simulink model "PIL_NO_RPI_new"  (R2021a)
settings: Solver=FixedStepAuto  StartTime=0.0  StopTime=60  FixedStep=0.001  RelTol=1e-3  EnableMultiTasking=on
values from neighbouring files (symbols this model uses):
  den_lpf_d = den_lpf20    [Mainframe_init.m]    (also in load_autopilot.m)
  Enable_Gyros = 0    [Mainframe_init.m]
  Enable_INS = 0    [Mainframe_init.m]
  num_lpf_d = num_lpf20    [Mainframe_init.m]    (also in load_autopilot.m)
undefined symbols (not defined in the file or in its folder): act_dmp, act_omega, Actuator, Aerodynamics, aMode, Autopilot, AUX, c_b_WGS, c_be, c_flat, c_grav, c_h_geop0, c_h_geope, c_pa0, c_pe, c_r0, c_rot, c_rsma, c_Tmp0, d_siB_0, d_siB_max, d_siB_min, dd_siB_max, dd_siB_min, dev, DiscIntNeverNeededParam, e_pa, e_Tmp, fin_maxrate, flag_I_act_switch, flag_I_aero_switch, flag_I_flat, flag_I_gravity_switch, flag_I_rot, h_bkpts_m, hcr, HIL_Data, JMMM_0, JMMM_e, JSPB_e, Ki_phi_vec, Kp_p_vec, Kp_phi_vec, lat_0, lon_0, Mass_Props, mB_0, mM_0, mM_e, National_Instruments, Newton, p, pBII_0, PCIe, phi, pMPB, pNPB, propellant_kg, prp_FBPB, prp_mdot ... (+40)
libraries: simulink x32, simulink_extras x23, aerolibcommonsys x4, pil_lib x2, custom_blocks x1, px4lib x1, sldrtlib x1, aerolibnav x1
(part 2 of 16)

== system PIL_NO_RPI_new/Servos1/Emulated Servos ==
  FCC Data : Inport
  Bus Creator : BusCreator  Inputs=4
  Bus Selector : BusSelector  OutputSignals=Control Surface Cmd.Fin_1_Cmd_rad,Control Surface Cmd.Fin_2_Cmd_rad,Control Surface Cmd.Fin_3_Cmd_rad,Control Surface Cmd.Fin_4_Cmd_rad
  Transfer Fcn{1..4} (4 alike) : TransferFcn  Numerator=33770  Denominator=[1 395.7 33770]
  Fin Deflections : Outport
  wires:
  FCC Data/1 -> Bus Selector/1
  Bus Selector/1 -> Transfer Fcn1/1  "<Fin_1_Cmd_rad>"
  Bus Selector/2 -> Transfer Fcn2/1  "<Fin_2_Cmd_rad>"
  Bus Selector/3 -> Transfer Fcn3/1  "<Fin_3_Cmd_rad>"
  Bus Selector/4 -> Transfer Fcn4/1  "<Fin_4_Cmd_rad>"
  Bus Creator/1 -> Fin Deflections/1
  Transfer Fcn1/1 -> Bus Creator/1  "Fin_1"
  Transfer Fcn2/1 -> Bus Creator/2  "Fin_2"
  Transfer Fcn3/1 -> Bus Creator/3  "Fin_3"
  Transfer Fcn4/1 -> Bus Creator/4  "Fin_4"

== system PIL_NO_RPI_new/Servos1/Real Servos ==
  FCC Data : Inport
  Bus Creator : BusCreator  Inputs=4
  Demux : Demux
  Encoder Input : sldrtlib/Encoder Input  SampleTime=0.001  MaxMissedTicks=10  ShowMissedTicks=off  YieldWhenWaiting=off  DrvName=National_Instruments/PCIe-6321  DrvAddress=4294967295  DrvOptions=[0 0 0 2 2 2 2]  Channels=1:4  QuadMode=3  IndexPulse=1  InputFilter=Inf  DataType=1
      settings: AttributesFormatString=National Instruments\nPCIe-6321 [auto]
  Reset Encoders : Subsystem
  Terminator : Terminator
  Ticks to rads : Gain  Gain=2*pi/4096
  Fin Deflections : Outport
  wires:
  Encoder Input/1 -> Ticks to rads/1
  FCC Data/1 -> Terminator/1
  Bus Creator/1 -> Fin Deflections/1
  Demux/3 -> Bus Creator/3  "Fin_3"
  Demux/2 -> Bus Creator/2  "Fin_2"
  Demux/1 -> Bus Creator/1  "Fin_1"
  Demux/4 -> Bus Creator/4  "Fin_4"
  [HIL_Ready] -> Reset Encoders/1(Reset Encoders)
  Ticks to rads/1 -> Reset Encoders/2(Encoder Readings)
  Reset Encoders/1(Fin Angles) -> Demux/1

== system PIL_NO_RPI_new/Virtual IMU/Gravity Vector ==
  Phi : Inport
  Theta : Inport  Port=2
  Cos : Trigonometry
  Cos1 : Trigonometry
  Cos2 : Trigonometry  Operator=cos
  Cos3 : Trigonometry  Operator=cos
  Multiply : Gain  Gain=9.81
  Multiply1 : Gain  Gain=9.81
  Multiply2 : Gain  Gain=-9.81
  Product : Product
  Product1 : Product
  Vector Concatenate1 : Concatenate  NumInputs=3
  g : Outport
  wires:
  Vector Concatenate1/1 -> g/1
  Cos/1 -> Multiply2/1
  Product/1 -> Multiply/1
  Cos1/1 -> Product/1
  Theta/1 -> Cos/1, Cos2/1
  Multiply/1 -> Vector Concatenate1/2
  Phi/1 -> Cos3/1, Cos1/1
  Product1/1 -> Multiply1/1
  Multiply1/1 -> Vector Concatenate1/3
  Multiply2/1 -> Vector Concatenate1/1
  Cos2/1 -> Product1/1, Product/2
  Cos3/1 -> Product1/2

== system PIL_NO_RPI_new/Flight Control Computer1/Communication Delay - 7ms/Triggered Subsystem ==
  In1 : Inport
  Trigger : TriggerPort  VariantControl=Variant
  Out1 : Outport
  wires:
  In1/1 -> Out1/1

== system PIL_NO_RPI_new/Flight Control Computer1/Communication Delay - 7ms1/Triggered Subsystem ==
  In1 : Inport
  Trigger : TriggerPort  VariantControl=Variant
  Out1 : Outport
  wires:
  In1/1 -> Out1/1

== system PIL_NO_RPI_new/Flight Control Computer1/PixBlock/Emulated Pixhawk1 ==
  Serial In : Inport
  Trigger : TriggerPort  VariantControl=Variant  PortDimensions=1
  Autopilot : Subsystem
  Convert to Bus : Subsystem
  Convert to Vector : Subsystem
  Fin Allocation : Subsystem
  IMU - Merge : Subsystem
  Inertial Navigation System : Subsystem
  Real Gyro : Subsystem
  Servo Commands : Subsystem  Commented=on
  Terminator : Terminator
  Zero : Constant  Value=0  OutDataTypeStr=Inherit: Inherit via back propagation
  Serial Out : Outport
  tag scope: Heartbeat=global
  wires:
  [Real_Gyro_Data] -> Convert to Vector/4(Real Gyro Data)
  Convert to Bus/2(Ext. Commands) -> [Ext_Cmd]
  Autopilot/1(Attitude_Commands) -> Fin Allocation/1(Attitude Cmd)  "ATT_Cmd"
  Convert to Bus/3(Enable INS Flag) -> Inertial Navigation System/1(Enable INS Flag)
  Inertial Navigation System/1(INS Data) -> [INS_Data]
  Zero/1 -> Convert to Vector/5(Debug Port)
  [Ext_Cmd] -> Autopilot/1(Cmd)
  [Heartbeat] -> Convert to Vector/2(Heartbeat)
  [IMU_Data] -> Autopilot/2(IMU Data)
  [INS_Data] -> Autopilot/3(INS Data)
  Convert to Bus/6(Virtual IMU Data) -> Real Gyro/1(HIL Gyro), IMU - Merge/1(HIL IMU)
  IMU - Merge/1(IMU Data) -> [IMU_Data], Inertial Navigation System/3(IMU Data)
  Convert to Vector/1(To HIL) -> Serial Out/1
  Fin Allocation/1(Fin Cmd) -> Servo Commands/1(Fin Cmd), Convert to Vector/1(Fin Deflections)
  Serial In/1 -> Convert to Bus/1(Input)
  [INS_Data] -> Convert to Vector/3(INS Data)
  Convert to Bus/4(Missile States) -> Inertial Navigation System/2(Missile States)
  Convert to Bus/1(Heartbeat) -> [Heartbeat]
  Convert to Bus/5(Real Gyros Flag) -> Terminator/1
  Real Gyro/1(Gyro Data) -> [Real_Gyro_Data]

== system PIL_NO_RPI_new/Flight Control Computer1/PixBlock1/__InputSSForSFun__ ==
  Serial In : Inport
  __UniqueOutportName__1__ : Outport
  wires:
  Serial In/1 -> __UniqueOutportName__1__/1

== system PIL_NO_RPI_new/Flight Control Computer1/PixBlock1/__OutputSSForSFun__ ==
  __UniqueInportName__1__ : Inport
  Serial Out : Outport
  wires:
  __UniqueInportName__1__/1 -> Serial Out/1

== system PIL_NO_RPI_new/Flight Control Computer1/Send to FCC/Heartbeat Counter ==
  note: Starting the heartbeat at negative values prevents unwanted FCC behaviour on startup
  Cast To Double14 : DataTypeConversion  OutDataTypeStr=single
  Heartbeat : simulink/Sources/Counter Free-Running  NumBits=16  tsamp=-1
  Subtract : Sum  Inputs=+-
  Zero : Constant  Value=1000  OutDataTypeStr=Inherit: Inherit via back propagation
  Out1 : Outport
  wires:
  Heartbeat/1 -> Cast To Double14/1
  Zero/1 -> Subtract/2
  Cast To Double14/1 -> Subtract/1  "send"
  Subtract/1 -> Out1/1

== system PIL_NO_RPI_new/Flight Control Computer2/Communication Delay - 7ms/Triggered Subsystem ==
  In1 : Inport
  Trigger : TriggerPort  VariantControl=Variant
  Out1 : Outport
  wires:
  In1/1 -> Out1/1

== system PIL_NO_RPI_new/Flight Control Computer2/Communication Delay - 7ms1/Triggered Subsystem ==
  In1 : Inport
  Trigger : TriggerPort  VariantControl=Variant
  Out1 : Outport
  wires:
  In1/1 -> Out1/1

== system PIL_NO_RPI_new/Flight Control Computer2/Communication Delay - 7ms2/Triggered Subsystem ==
  In1 : Inport
  Trigger : TriggerPort  VariantControl=Variant
  Out1 : Outport
  wires:
  In1/1 -> Out1/1

== system PIL_NO_RPI_new/Flight Control Computer2/Pixhawk1/FCC Logic1 ==
  Ext. Commands : Inport
  FDM States : Inport  Port=2
  ALT : Inport  Port=3
  Control : Subsystem
  Fin Allocation : Subsystem
  variable switch : Subsystem
  Fin Deflections : Outport
  wires:
  Fin Allocation/1(siB_cmd) -> Fin Deflections/1
  Control/1(Attitude_Commands) -> Fin Allocation/1(Input1)  "ATT_Cmd"
  Ext. Commands/1 -> Control/1(cmd)
  variable switch/1(State Bus) -> Control/2(states)
  FDM States/1 -> variable switch/1(Simulation States)
  ALT/1 -> Control/3(ALT)

== system PIL_NO_RPI_new/Flight Control Computer2/Pixhawk1/Send to HIL ==
  Fin Deflections1 : Inport
  Heartbeat1 : Inport  Port=2
  Debug Port1 : Inport  Port=3
  Cast To Single : DataTypeConversion  OutDataTypeStr=single
  Cast To Single3 : DataTypeConversion  OutDataTypeStr=single
  Cast To Single4 : DataTypeConversion  OutDataTypeStr=single
  Demux1 : Demux
  Vector Concatenate1 : Concatenate  NumInputs=6
  control_allocation1 : Subsystem
  Data Out : Outport
  wires:
  Cast To Single/1 -> Data Out/1
  Heartbeat1/1 -> Vector Concatenate1/1
  control_allocation1/1(siB_cmd) -> Cast To Single4/1
  Fin Deflections1/1 -> Cast To Single3/1
  Cast To Single3/1 -> control_allocation1/1(fin_cmd)
  Cast To Single4/1 -> Demux1/1
  Demux1/1 -> Vector Concatenate1/2  "siB_cmd_1"
  Demux1/2 -> Vector Concatenate1/3  "siB_cmd_2"
  Demux1/3 -> Vector Concatenate1/4  "siB_cmd_3"
  Demux1/4 -> Vector Concatenate1/5  "siB_cmd_4"
  Debug Port1/1 -> Vector Concatenate1/6
  Vector Concatenate1/1 -> Cast To Single/1

== system PIL_NO_RPI_new/Flight Control Computer2/Pixhawk1/data2bus ==
  raw_data : Inport  OutDataTypeStr=single
  Bus Creator : BusCreator  Inputs=9
  Bus Creator1 : BusCreator  Inputs=1
  Demux : Demux  Outputs=13
  Ext. Commands : Outport  OutDataTypeStr=single
  FDM States : Outport  Port=2  OutDataTypeStr=single
  Heartbeat : Outport  Port=3
  FCC Enabled : Outport  Port=4
  Use Sim States : Outport  Port=5
  wires:
  Demux/10 -> Bus Creator/7  "u"
  Demux/3 -> Use Sim States/1  "Use Sim States"
  Demux/2 -> Heartbeat/1  "Hearbeat"
  Demux/8 -> Bus Creator/5  "q"
  Demux/4 -> Bus Creator/1  "phi"
  Demux/5 -> Bus Creator/2  "theta"
  Demux/7 -> Bus Creator/4  "p"
  Demux/9 -> Bus Creator/6  "r"
  Demux/6 -> Bus Creator/3  "psi"
  Demux/13 -> Bus Creator1/1  "phi_cmd"
  Demux/12 -> Bus Creator/9  "w"
  Demux/11 -> Bus Creator/8  "v"
  raw_data/1 -> Demux/1
  Bus Creator/1 -> FDM States/1
  Bus Creator1/1 -> Ext. Commands/1
  Demux/1 -> FCC Enabled/1  "EnableFCC"

== system PIL_NO_RPI_new/Flight Control Computer2/Pixhawk2/__InputSSForSFun__ ==
  Input Data : Inport
  "ALT " : Inport  Port=2
  __UniqueOutportName__1__ : Outport
  __UniqueOutportName__2__ : Outport  Port=2
  wires:
  "ALT "/1 -> __UniqueOutportName__2__/1
  Input Data/1 -> __UniqueOutportName__1__/1

== system PIL_NO_RPI_new/Flight Control Computer2/Pixhawk2/__OutputSSForSFun__ ==
  __UniqueInportName__1__ : Inport
  Output Data : Outport
  wires:
  __UniqueInportName__1__/1 -> Output Data/1

== system PIL_NO_RPI_new/Flight Control Computer2/Send to Pixhawk/HeartBeat ==
  note: Starting the heartbeat at negative values prevents unwanted FCC behaviour on startup
  Cast To Double14 : DataTypeConversion  OutDataTypeStr=single
  Heartbeat : simulink/Sources/Counter Free-Running  NumBits=16  tsamp=-1
  Subtract : Sum  Inputs=+-
  Zero : Constant  Value=1000  OutDataTypeStr=Inherit: Inherit via back propagation
  Out1 : Outport
  wires:
  Heartbeat/1 -> Cast To Double14/1
  Zero/1 -> Subtract/2
  Cast To Double14/1 -> Subtract/1  "send"
  Subtract/1 -> Out1/1

== system PIL_NO_RPI_new/Flight Control Computer2/Send to Pixhawk/State Mixer ==
  States : Inport
  Bus Selector : BusSelector  OutputSignals=Attitude_States.ATT_Euler.Phi_rad,Attitude_States.ATT_Euler.Theta_rad,Attitude_States.ATT_Euler.Psi_rad,Rotation_States.p_radDs,Rotation_States.q_radDs,Rotation_States.r_radDs,Translation_States.u_mDs,Translation_States.v_mDs,Translation_States.w_mDs
  Phi_rad : Outport
  Theta_rad : Outport  Port=2
  Psi_rad : Outport  Port=3
  p_radDs : Outport  Port=4
  q_radDs : Outport  Port=5
  r_radDs : Outport  Port=6
  u_mDs : Outport  Port=7
  v_mDs : Outport  Port=8
  w_mDs : Outport  Port=9
  wires:
  Bus Selector/3 -> Psi_rad/1  "<Psi_rad>"
  Bus Selector/9 -> w_mDs/1  "<w_mDs>"
  Bus Selector/1 -> Phi_rad/1  "<Phi_rad>"
  Bus Selector/5 -> q_radDs/1  "<q_radDs>"
  Bus Selector/7 -> u_mDs/1  "<u_mDs>"
  Bus Selector/6 -> r_radDs/1  "<r_radDs>"
  Bus Selector/2 -> Theta_rad/1  "<Theta_rad>"
  States/1 -> Bus Selector/1
  Bus Selector/8 -> v_mDs/1  "<v_mDs>"
  Bus Selector/4 -> p_radDs/1  "<p_radDs>"

== system PIL_NO_RPI_new/Flight Gear Simulator/Flight Simulator On/Flat Earth to LLA ==
  Xe : Inport  Unit=m
  ground height : Inport  Port=2  Unit=m
  Disallow CGS : UnitConfiguration  UnitSystemsStr=English,SI,SI (extended)  AllowAllUnitSystems=off
  LatLong wrap : Subsystem
      mask init:
      | aeroicon('aeroblk')
      mask Display:
      | port_label('input',1,'[\mu l]','texmode','on')
      | port_label('output',1,'[\mu l]_{wrap}','texmode','on')
  LatLong wrap1 : Subsystem
      mask init:
      | aeroicon('aeroblk')
      mask Display:
      | port_label('input',1,'[\mu l]','texmode','on')
      | port_label('output',1,'[\mu l]_{wrap}','texmode','on')
  LongLat_offset : Subsystem
  Sel1 : Selector  InputPortWidth=3  IndexOptions=Index vector (dialog)  Indices=[1,2]  OutputSizes=1
  Sel2 : Selector  InputPortWidth=3  IndexOptions=Index vector (dialog)  Indices=3  OutputSizes=1
  Sum : Sum  Inputs=|++
  Sum1 : Sum  Inputs=-+
  "Xe " : InportShadow  Unit=m
  Ze2height : UnaryMinus
  initial_latg : Selector  InputPortWidth=2  IndexOptions=Index vector (dialog)  Indices=[1]  OutputSizes=1
  initial_pos : Constant  Value=LL0
  pos_deg : Subsystem
  mu l : Outport  Unit=deg  VectorParamsAs1DForOutWhenUnconnected=off
  h : Outport  Port=2  Unit=m  VectorParamsAs1DForOutWhenUnconnected=off
  wires:
  pos_deg/1(out) -> Sum/1
  LongLat_offset/1(DeltaLL_rad) -> pos_deg/1(in)
  LatLong wrap1/1(Lat/Long wrapped) -> initial_latg/1, Sum/2
  initial_pos/1 -> LatLong wrap1/1(LatLong)
  LatLong wrap/1(Lat/Long wrapped) -> mu l/1
  initial_latg/1 -> LongLat_offset/2(mu)
  "Xe "/1 -> Sel2/1
  Sel1/1 -> LongLat_offset/1(XY)
  ground height/1 -> Sum1/1
  Sum1/1 -> h/1
  Ze2height/1 -> Sum1/2  "alt"
  Sel2/1 -> Ze2height/1
  Sum/1 -> LatLong wrap/1(LatLong)
  Xe/1 -> Sel1/1

== system PIL_NO_RPI_new/Flight Gear Simulator/Flight Simulator On/FlightGear Preconfigured 6DoF Animation ==
  In1 : Inport
  Angle Conversion : Subsystem
  Angle Conversion1 : Subsystem
  Demux : Demux  Outputs=6
  Pack net_fdm Packet for FlightGear : S-Function  FunctionName=saerofgpacknetfdm  Parameters=packetVersion, 'on','off','off','off','off','off', SampleTime  SFunctionDeploymentMode=off  EnableBusSupport=off
  PacketSize : Constant  Value=408
  Rate Transition : RateTransition  Integrity=off  Deterministic=off  OutPortSampleTime=SampleTime
  Simulation Pace : S-Function  FunctionName=saeroclockpacer  Parameters=SimulationPace,SleepMode,OutputPaceError,SampleTime  SFunctionDeploymentMode=off  EnableBusSupport=off  mask(Simulation Pace){SimulationPace=1, SleepMode=MATLAB Thread, OutputPaceError=off, SampleTime=SampleTime}
      mask prompts: SimulationPace "aeroblks:aeroblkanimutils:blockSimulationPaceParamSimulationpacesimsecperclocksec"; SleepMode "aeroblks:aeroblkanimutils:blockSimulationPaceParamSleepmode"; OutputPaceError "aeroblks:aeroblkanimutils:blockSimulationPaceParamOutputpaceerrorsec"; SampleTime "aeroblks:aeroblkanimutils:blockSimulationPaceParamSampletime1forinherited"
      mask help: aeroblks:aeroblkanimutils:blockSimulationPaceDesc
      mask init:
      | aeroicon('aeroblkpacer');
      settings: AttributesFormatString=%<SimulationPace> sec/sec
      mask Help: eval('asbhelp');
      mask TypeOptions SleepMode: aeroblks:aeroblkanimutils:blockSimulationPaceParamComboOff | aeroblks:aeroblkanimutils:blockSimulationPaceParamComboMATLABThread | aeroblks:aeroblkanimutils:blockSimulationPaceParamComboBusyWait | aeroblks:aeroblkanimutils:blockSimulationPaceParamComboAuto
      mask DialogControl SimulationPace Prompt: Simulation pace (sim sec per clock sec):
      mask DialogControl SleepMode Prompt: Sleep mode:
      mask DialogControl OutputPaceError Prompt: Output pace error (sec)
      mask DialogControl SampleTime Prompt: Sample time (-1 for inherited):
      mask Display:
      | text(0.5,0.60,'Set','horizontalAlignment','center');
      | text(0.5,0.40,'Pace','horizontalAlignment','center');
  UDP Send : S-Function  FunctionName=saerofgsend  Parameters=DestinationIpAddress,DestinationPort,-1,SampleTime,0  SFunctionDeploymentMode=off  EnableBusSupport=off
  Unit Sys : UnitConfiguration  UnitSystemsStr=SI,SI (extended)  AllowAllUnitSystems=off
  toSingle1 : DataTypeConversion  OutDataTypeStr=single
  toSingle2 : DataTypeConversion  OutDataTypeStr=single
  toSingle3 : DataTypeConversion  OutDataTypeStr=single
  wires:
  Angle Conversion1/1(out) -> Pack net_fdm Packet for FlightGear/2
  Angle Conversion/1(out) -> Pack net_fdm Packet for FlightGear/1
  Rate Transition/1 -> Demux/1
  toSingle3/1 -> Pack net_fdm Packet for FlightGear/6
  toSingle2/1 -> Pack net_fdm Packet for FlightGear/5
  toSingle1/1 -> Pack net_fdm Packet for FlightGear/4
  Pack net_fdm Packet for FlightGear/1 -> UDP Send/1
  In1/1 -> Rate Transition/1
  Demux/1 -> Angle Conversion/1(in)
  Demux/2 -> Angle Conversion1/1(in)
  Demux/3 -> Pack net_fdm Packet for FlightGear/3
  Demux/4 -> toSingle1/1
  Demux/5 -> toSingle2/1
  Demux/6 -> toSingle3/1
  PacketSize/1 -> UDP Send/2

== system PIL_NO_RPI_new/Flight Gear Simulator/Flight Simulator On/FlightGear1 ==

== system PIL_NO_RPI_new/Non-linear Flight Dynamic Model1/Environment/Enabled Subsystem1 ==
  Enable : EnablePort
  Digital Clock : DigitalClock  SampleTime=-1
  CalibrationTime : Outport  InitialOutput=0
  wires:
  Digital Clock/1 -> CalibrationTime/1

== system PIL_NO_RPI_new/Non-linear Flight Dynamic Model1/Environment/atm_dynamic ==
  Add : Sum
  Add1 : Sum
  Bus Creator : BusCreator  Inputs=1
  Constant1 : Constant  Value=0
  Vector Concatenate : Concatenate  NumInputs=3
  course_angle_uncertainty : Constant  Value=0
  course_angle_wind : Constant  Value=0
  trafo_around_z_axis : Subsystem  mask(Transformation um z-Achse){}
      mask help: Dieser Block transformiert einen Vektor vec1 durch eine Drehung des Referenzkoordinatensystems um die z-Achse und um den Winkel gamma (in rad) in den Vektor vec2
      mask Help:
      | Name:
      | 
      |    trafo_around_z_axis
      | 
      | Beschreibung:
      | 
      |    Dieser Block transformiert einen Vektor vec1 durch eine Drehung des
      |    Referenzkoordinatensystems um die z-Achse und um den Winkel gamma
      |    (in rad) in den Vektor vec2
      | 
      | Inputs   [dimension]  [data type] [unit]:
      | 
      |     vec1    [3] [double] [-]
      |     gamma   [1] [double] [rad]
      | 
      | Outputs  [dimension]  [data type] [unit]:
      | 
      |     vec2  [3] [double] [-]
  vWW : Constant  Value=0
  vWW_uncertainty : Constant  Value=0
  vWEG : Outport  VectorParamsAs1DForOutWhenUnconnected=off
  wires:
  Bus Creator/1 -> vWEG/1  "atm_dyn_bus"
  trafo_around_z_axis/1(vec2) -> Bus Creator/1  "vWEG"
  Add1/1 -> Vector Concatenate/1
  course_angle_uncertainty/1 -> Add/2
  Constant1/1 -> Vector Concatenate/2, Vector Concatenate/3
  vWW/1 -> Add1/2
  Vector Concatenate/1 -> trafo_around_z_axis/1(vec1)
  Add/1 -> trafo_around_z_axis/2(gamma)
  vWW_uncertainty/1 -> Add1/1
  course_angle_wind/1 -> Add/1

== system PIL_NO_RPI_new/Non-linear Flight Dynamic Model1/Extract States/Assemble_States_Bus1 ==
  Translation_States : Inport
  Rotation_States : Inport  Port=2
  Translation_States_Dot : Inport  Port=3
  Rotation_States_Dot : Inport  Port=4
  Attitude_States : Inport  Port=5
  POS_NED : Inport  Port=6
  POS_NED_dot : Inport  Port=7
  Bus Creator{1,4..6,8,12..13} (7 alike) : BusCreator  Inputs=3
  Bus Creator3 : BusCreator  Inputs=7
  Bus Creator7 : BusCreator  Inputs=2
  Bus Creator9 : BusCreator  Inputs=4
  Demux : Demux
  Demux{1..7} (7 alike) : Demux  Outputs=3
  Rotation Angles to Quaternions : Subsystem  mask(Ang2Quat){rotationOrder=ZYX, aMode=aMode}
      mask prompts: rotationOrder "shared_aeroblks:sharedaeroblktransform:blockAng2QuatParamRotationOrder"
      mask help: shared_aeroblks:sharedaeroblktransform:blockAng2QuatDesc
      mask init:
      | if aerosharedtest(gcb)
      |     ports=aerosharedicon('sharedang2quat');
      | else
      |     ports=sharedautoicon('sharedang2quat');
      | end
      settings: AttributesFormatString=Rotation Order: %<rotationOrder>
      mask Help: eval('if license(''test'',''Aerospace_Blockset'')aerosharedhelp(''rotation_angles_to_quaternions'');elseif license(''test'',''Powertrain_Blockset'')sharedautohelp(''rotation_angles_to_quaternions'');end')
      mask TypeOptions rotationOrder: shared_aeroblks:sharedaeroblktransform:blockParamComboZYX | shared_aeroblks:sharedaeroblktransform:blockParamComboZYZ | shared_aeroblks:sharedaeroblktransform:blockParamComboZXY | shared_aeroblks:sharedaeroblktransform:blockParamComboZXZ | shared_aeroblks:sharedaeroblktransform:blockParamComboYXZ | shared_aeroblks:sharedaeroblktransform:blockParamComboYXY | shared_aeroblks:sharedaeroblktransform:blockParamComboYZX | shared_aeroblks:sharedaeroblktransform:blockParamComboYZY | shared_aeroblks:sharedaeroblktransform:blockParamComboXYZ | shared_aeroblks:sharedaeroblktransform:blockParamComboXYX | shared_aeroblks:sharedaeroblktransform:blockParamComboXZY | shared_aeroblks:sharedaeroblktransform:blockParamComboXZX
      mask DialogControl rotationOrder Prompt: Rotation order:
      mask Display:
      | port_label('input',1,'[R_1,R_2,R_3]','texmode','on')
      | port_label('output',1,'q','texmode','on')
  Selector : Selector  InputPortWidth=3  IndexOptions=Index vector (dialog)  Indices=[3,2,1]  OutputSizes=1
  Three-axis Inertial Measurement Unit3 : Subsystem  Commented=on  mask(Three-axis Inertial Measurement Unit){units=Metric (MKS), imu=[0 0 0], i_Ts=0, dtype_a=on, w_a=190, z_a=0.707, a_sf_cc=[1 0 0; 0 1 0; 0 0 1], a_bias=[0 0 0], a_sat=[-inf  -inf  -inf  inf inf inf], dtype_g=on, w_g=190, z_g=0.707, g_sf_cc=[1 0 0; 0 1 0; 0 0 1], g_bias=[0 0 0], g_sens=[0 0 0], g_sat=[-inf  -inf  -inf  inf inf inf], i_rand=on, i_seeds=[23093 23094 23095 23096 23097 23098], i_pow=[0.001 0.001 0.001 0.0001 0.0001 0.0001]}
      mask prompts: units "aeroblks:aeroblknav:blockThreeaxisInertialMeasurementUnitParamUnits"; imu "aeroblks:aeroblknav:blockThreeaxisInertialMeasurementUnitParamIMUlocation"; i_Ts "aeroblks:aeroblknav:blockThreeaxisInertialMeasurementUnitParamUpdaterate"; dtype_a "aeroblks:aeroblknav:blockThreeaxisInertialMeasurementUnitParamSecondorderdynamicsforaccelerometer"; w_a "aeroblks:aeroblknav:blockThreeaxisInertialMeasurementUnitParamAccelerometernaturalfrequencyradsec"; z_a "aeroblks:aeroblknav:blockThreeaxisInertialMeasurementUnitParamAccelerometerdampingratio"; a_sf_cc "aeroblks:aeroblknav:blockThreeaxisInertialMeasurementUnitParamAccelerometerscalefactorandcrosscoupling"; a_bias "aeroblks:aeroblknav:blockThreeaxisInertialMeasurementUnitParamAccelerometermeasurementbias"; a_sat "aeroblks:aeroblknav:blockThreeaxisInertialMeasurementUnitParamAccelerometerupperandlowerlimits"; dtype_g "aeroblks:aeroblknav:blockThreeaxisInertialMeasurementUnitParamSecondorderdynamicsforgyro"; w_g "aeroblks:aeroblknav:blockThreeaxisInertialMeasurementUnitParamGyronaturalfrequencyradsec"; z_g "aeroblks:aeroblknav:blockThreeaxisInertialMeasurementUnitParamGyrodampingratio"; g_sf_cc "aeroblks:aeroblknav:blockThreeaxisInertialMeasurementUnitParamGyroscalefactorsandcrosscoupling"; g_bias "aeroblks:aeroblknav:blockThreeaxisInertialMeasurementUnitParamGyromeasurementbias"; g_sens "aeroblks:aeroblknav:blockThreeaxisInertialMeasurementUnitParamGsensitivebias"; g_sat "aeroblks:aeroblknav:blockThreeaxisInertialMeasurementUnitParamGyroupperandlowerlimits"; i_rand "aeroblks:aeroblknav:blockThreeaxisInertialMeasurementUnitParamNoiseon"; i_seeds "aeroblks:aeroblknav:blockThreeaxisInertialMeasurementUnitParamNoiseseeds"; i_pow "aeroblks:aeroblknav:blockThreeaxisInertialMeasurementUnitParamNoisepower"
      mask help: aeroblks:aeroblknav:blockThreeaxisInertialMeasurementUnitDesc
      mask init:
      | block = gcb;   
      | ports=aeroicon('aeroblkimu','icon');
      mask Help: eval('asbhelp');
      mask TypeOptions units: aeroblks:aeroblknav:blockThreeaxisInertialMeasurementUnitParamComboMetricMKS | aeroblks:aeroblknav:blockThreeaxisInertialMeasurementUnitParamComboEnglish
      mask Callback dtype_a: aeroicon('aeroblkimu')
      mask Callback dtype_g: aeroicon('aeroblkimu')
      mask Callback i_rand: aeroicon('aeroblkimu')
      mask DialogControl ParameterTabVar0 Prompt: Main
      mask DialogControl units Prompt: Units:
      mask DialogControl imu Prompt: IMU location:
      mask DialogControl i_Ts Prompt: Update rate:
      mask DialogControl ParameterTabVar01 Prompt: Accelerometer
      mask DialogControl dtype_a Prompt: Second-order dynamics for accelerometer
      mask DialogControl w_a Prompt: Accelerometer natural frequency (rad/sec):
      mask DialogControl z_a Prompt: Accelerometer damping ratio:
      mask DialogControl a_sf_cc Prompt: Accelerometer scale factor and cross-coupling:
      mask DialogControl a_bias Prompt: Accelerometer measurement bias:
      mask DialogControl a_sat Prompt: Accelerometer upper and lower limits:
      mask DialogControl ParameterTabVar012 Prompt: Gyroscope
      mask DialogControl dtype_g Prompt: Second-order dynamics for gyro
      mask DialogControl w_g Prompt: Gyro natural frequency (rad/sec):
      mask DialogControl z_g Prompt: Gyro damping ratio:
      mask DialogControl g_sf_cc Prompt: Gyro scale factors and cross-coupling:
      mask DialogControl g_bias Prompt: Gyro measurement bias:
      mask DialogControl g_sens Prompt: G-sensitive bias:
      mask DialogControl g_sat Prompt: Gyro upper and lower limits:
      mask DialogControl ParameterTabVar0123 Prompt: Noise
      mask DialogControl i_rand Prompt: Noise on
      mask DialogControl i_seeds Prompt: Noise seeds:
      mask DialogControl i_pow Prompt: Noise power:
      mask Display:
      | port_label(ports(1).type,ports(1).port,ports(1).txt,'texmode','on');
      | port_label(ports(2).type,ports(2).port,ports(2).txt,'texmode','on');
      | port_label(ports(3).type,ports(3).port,ports(3).txt,'texmode','on');
      | port_label(ports(4).type,ports(4).port,ports(4).txt,'texmode','on');
      | port_label(ports(5).type,ports(5).port,ports(5).txt,'texmode','on');
      | port_label(ports(6).type,ports(6).port,ports(6).txt,'texmode','on');
      | port_label(ports(7).type,ports(7).port,ports(7).txt,'texmode','on');
  States : Outport  VectorParamsAs1DForOutWhenUnconnected=off
  wires:
  Bus Creator7/1 -> Bus Creator3/5  "Attitude_States"
  Demux/3 -> Bus Creator9/3  "quat_2"
  Demux/4 -> Bus Creator9/4  "quat_3"
  Demux/1 -> Bus Creator9/1  "quat_0"
  Bus Creator9/1 -> Bus Creator7/2  "ATT_Quaternions"
  Bus Creator12/1 -> Bus Creator3/6  "POS_NED"
  Demux/2 -> Bus Creator9/2  "quat_1"
  Bus Creator8/1 -> Bus Creator7/1  "ATT_Euler"
  Bus Creator4/1 -> Bus Creator3/1  "Translation_States"
  Bus Creator6/1 -> Bus Creator3/2  "Rotation_States"
  Bus Creator5/1 -> Bus Creator3/3  "Translation_States_Dot"
  Rotation Angles to Quaternions/1(Quat) -> Demux/1
  Demux6/3 -> Bus Creator12/3  "POS_z_NED_m"
  Demux6/2 -> Bus Creator12/2  "POS_y_NED_m"
  Demux6/1 -> Bus Creator12/1  "POS_x_NED_m"
  Demux5/3 -> Bus Creator8/3  "Psi_rad"
  Demux5/2 -> Bus Creator8/2  "Theta_rad"
  Demux5/1 -> Bus Creator8/1  "Phi_rad"
  Demux2/3 -> Bus Creator6/3  "r_radDs"
  Demux2/2 -> Bus Creator6/2  "q_radDs"
  Demux2/1 -> Bus Creator6/1  "p_radDs"
  Demux3/3 -> Bus Creator5/3  "w_dot_mDs2"
  Demux3/2 -> Bus Creator5/2  "v_dot_mDs2"
  Demux3/1 -> Bus Creator5/1  "u_dot_mDs2"
  Demux1/3 -> Bus Creator4/3  "w_mDs"
  Demux1/2 -> Bus Creator4/2  "v_mDs"
  Demux1/1 -> Bus Creator4/1  "u_mDs"
  Bus Creator13/1 -> Bus Creator3/4  "Rotation_States_Dot"
  Demux4/1 -> Bus Creator13/1  "p_dot_radDs2"
  Demux4/2 -> Bus Creator13/2  "q_dot_radDs2"
  Demux4/3 -> Bus Creator13/3  "r_dot_radDs2"
  Translation_States/1 -> Demux1/1
  Rotation_States/1 -> Demux2/1
  Translation_States_Dot/1 -> Demux3/1
  Rotation_States_Dot/1 -> Demux4/1
  Attitude_States/1 -> Selector/1, Demux5/1
  POS_NED/1 -> Demux6/1
  Bus Creator3/1 -> States/1  "FDM_States"
  Selector/1 -> Rotation Angles to Quaternions/1("R1, R2, R3")
  POS_NED_dot/1 -> Demux7/1
  Demux7/2 -> Bus Creator1/2  "POS_y_NED_dot_m"
  Demux7/3 -> Bus Creator1/3  "POS_z_NED_dot_m"
  Bus Creator1/1 -> Bus Creator3/7  "POS_NED_dot"
  Demux7/1 -> Bus Creator1/1  "POS_x_NED_dot_m"

== system PIL_NO_RPI_new/Non-linear Flight Dynamic Model1/Extract States/quaternion_to_euler_angles1 ==
  note: Um numerische Probleme zu
      | vermeiden, wird hier eine Saturiierung
      | benutzt.
  note: Outputs [size]:
      |
      | roll angle [1]
      | pitch angle [1]
      | yaw angle [1]
  note: Inputs [size]:
      |
      | quaternion [4]
  q : Inport  PortDimensions=4
  Add : Sum
  Add1 : Sum  Inputs=+--
  Add2 : Sum  Inputs=+-
  Add3 : Sum
  Add4 : Sum  Inputs=+--
  Complex to Real-Imag : ComplexToRealImag  Output=Real
  Constant : Constant  Value=0.5
  Constant1 : Constant  Value=0.5
  Demux : Demux
  Gain : Gain  Gain=2
  Product{,1..9} (10 alike) : Product
  Saturation : Saturate  UpperLimit=1  LowerLimit=-1
      settings: AttributesFormatString=|
      | %<UpperLimit>
      | %<LowerLimit>
  Trigonometric Function : Trigonometry  Operator=atan2
  Trigonometric Function1 : Trigonometry  Operator=asin
  Trigonometric Function2 : Trigonometry  Operator=atan2
  Vector Concatenate : Concatenate  NumInputs=3
  eulx : Outport  VectorParamsAs1DForOutWhenUnconnected=off
  wires:
  Vector Concatenate/1 -> Complex to Real-Imag/1
  Complex to Real-Imag/1 -> eulx/1
  Trigonometric Function2/1 -> Vector Concatenate/3
  Trigonometric Function1/1 -> Vector Concatenate/2
  Trigonometric Function/1 -> Vector Concatenate/1
  Add/1 -> Trigonometric Function/1
  Product1/1 -> Add/2
  Product/1 -> Add/1
  Product3/1 -> Add1/3
  Product2/1 -> Add1/2
  Product5/1 -> Add2/2
  Product4/1 -> Add2/1
  Product7/1 -> Add3/2
  Product6/1 -> Add3/1
  Add3/1 -> Trigonometric Function2/1
  Add4/1 -> Trigonometric Function2/2
  Add2/1 -> Gain/1
  Add1/1 -> Trigonometric Function/2
  q/1 -> Demux/1
  Demux/4 -> Product7/2, Product4/2, Product/2  "4"
  Demux/1 -> Product2/2, Product2/1, Product/1, Product6/1, Product5/1  "1"
  Demux/2 -> Product4/1, Product3/2, Product3/1, Product1/1, Product8/2, Product8/1, Product6/2  "2"
  Constant/1 -> Add1/1
  Product9/1 -> Add4/3
  Product8/1 -> Add4/2
  Constant1/1 -> Add4/1
  Demux/3 -> Product9/2, Product9/1, Product7/1, Product1/2, Product5/2  "3"
  Gain/1 -> Saturation/1
  Saturation/1 -> Trigonometric Function1/1

== system PIL_NO_RPI_new/Non-linear Flight Dynamic Model1/GRM_Airframe/aerodynamics ==
  str_flow : Inport
  fin : Inport  Port=2
  wab : Inport  Port=3
  env_glbl : Inport  Port=4
  Bus Selector : BusSelector  OutputSignals=qdynB,MaB,alB,beB,hBE,wBIB_star
  Bus Selector1 : BusSelector  OutputSignals=afinB
  Bus Selector2 : BusSelector  OutputSignals=pBPB
  aerodynamic_via_lookup : Subsystem
  logic_base_drag : Subsystem
  aero : Outport  VectorParamsAs1DForOutWhenUnconnected=off
  wires:
  str_flow/1 -> Bus Selector/1
  wab/1 -> Bus Selector2/1
  fin/1 -> Bus Selector1/1
  Bus Selector2/1 -> aerodynamic_via_lookup/1(pBPB)  "<pBPB>"
  Bus Selector/1 -> aerodynamic_via_lookup/2(qdynB)  "<qdynB>"
  Bus Selector/2 -> aerodynamic_via_lookup/3(MaB)  "<MaB>"
  Bus Selector/3 -> aerodynamic_via_lookup/4(alB)  "<alB>"
  Bus Selector/4 -> aerodynamic_via_lookup/5(beB)  "<beB>"
  Bus Selector/5 -> aerodynamic_via_lookup/6(hBE)  "<hBE>"
  Bus Selector1/1 -> aerodynamic_via_lookup/8(afinB)  "<afinB>"
  Bus Selector/6 -> aerodynamic_via_lookup/7(wBIB_star)  "<wBIB_star>"
  aerodynamic_via_lookup/1(aero_bus) -> aero/1
  env_glbl/1 -> logic_base_drag/1(env_glbl)
  logic_base_drag/1(flag_base_drag) -> aerodynamic_via_lookup/9(flag_I_prp)

== system PIL_NO_RPI_new/Non-linear Flight Dynamic Model1/GRM_Airframe/environment ==
  flight_dyn : Inport
  env_glbl : Inport  Port=2
  Bus Creator1 : BusCreator  Inputs=2
  Bus Creator2 : BusCreator  Inputs=2
  Bus Selector : BusSelector  OutputSignals=lon,lat,hBE
  Bus Selector1 : BusSelector  OutputSignals=atm_dyn_bus
  Saturation : Saturate  UpperLimit=inf  LowerLimit=eps
      settings: AttributesFormatString=|
      | %<UpperLimit>
      | %<LowerLimit>
  WGS84_Gravitation : Subsystem  mask{flg_omega_enabled=on}
      mask prompts: flg_omega_enabled "Zentripetalbeschleunigung mitberechnen"
      mask help:
      | Dieser Block berechnet die Gravitation für das idealisierte WGS84
      | Ellipsoid. Die Berechnung ist hierbei nach dem Technical Report
      | "Department of Defense World Geodetic System 1984", NIMA TR8350.2,
      | Third Edition, Amendment 1 vom 3 Januar 2000 implementiert.
      | Das Modell ist gültig für alle Höhen über dem WGS84 Referenzellipsoid, und
      | ist somit der reinen Taylorexpansion des Somigliana Modells überlegen
      | (siehe Kapitel 4.3 des WGS84 reports).
      |
      | ---------------------------------------------------------------------------
      | Longitude [rad]: Nach WGS84 definierte Geodätische Länge.  (lambda)
      | Lattitude [rad]: Nach WGS84 definierte Geodätische Breite. (phi)
      | Height [m]: Höhe über dem WGS84 Referenzellipsoid.
      mask init:
      | [ c_rsma, c_b_WGS, c_grav, c_rot] = init_WGS84_Gravitationsmodell();
  atmosphere_static_ISO_2533 : Subsystem
  convert_to_local_frame : Subsystem
  env : Outport  VectorParamsAs1DForOutWhenUnconnected=off
  wires:
  convert_to_local_frame/1(gBG) -> Bus Creator2/1
  flight_dyn/1 -> Bus Selector/1
  WGS84_Gravitation/1(gE) -> convert_to_local_frame/1(gE)
  Bus Selector/1 -> WGS84_Gravitation/1(lon)  "<lon>"
  Bus Selector/3 -> atmosphere_static_ISO_2533/1(hBE), Saturation/1  "<hBE>"
  Bus Creator2/1 -> env/1  "env_bus"
  Bus Selector/2 -> WGS84_Gravitation/2(lat)  "<lat>"
  Bus Creator1/1 -> Bus Creator2/2  "atm_bus"
  Saturation/1 -> WGS84_Gravitation/3(h)
  atmosphere_static_ISO_2533/1(atm_stat) -> Bus Creator1/1  "atm_stat_bus"
  env_glbl/1 -> Bus Selector1/1, atmosphere_static_ISO_2533/2(env_glbl)
  Bus Selector1/1 -> Bus Creator1/2  "<atm_dyn_bus>"

== system PIL_NO_RPI_new/Non-linear Flight Dynamic Model1/GRM_Airframe/fin_actuators ==
  cmd : Inport
  Bus Creator3 : BusCreator  Inputs=7
  Bus Selector : BusSelector  OutputSignals=siB_cmd
  Constant : Constant  Value=flag_I_act_switch
  Constant7 : Constant  Value=tRRR
  Demux : Demux
  Rudder : Subsystem  mask{siB_max=siB_max, siB_min=siB_min, d_siB_max=d_siB_max, d_siB_min=d_siB_min, dd_siB_max=dd_siB_max, dd_siB_min=dd_siB_min, omega=act_omega, dmp=act_dmp, unc_bl=unc_act_bl, unc_scale=unc_act_scale, unc_off=unc_act_off, siB_0=siB_0, d_siB_0=d_siB_0}
      mask prompts: siB_max "Obere Limitierung des Ruderstellwinkels in [rad]"; siB_min "Untere Limitierung des Ruderstellwinkels in [rad]"; d_siB_max "Obere Limitierung der Ruderstellwinkelgeschwindigkeit in [rad/s]"; d_siB_min "Untere Limitierung der Ruderstellwinkelgeschwindigkeit in [rad/s]"; dd_siB_max "Obere Limitierung der Ruderstellwinkelbeschleunigung in [rad/s^2]"; dd_siB_min "Untere Limitierung der Ruderstellwinkelbeschleunigung in [rad/s^2]"; omega "Eckfrequenz in [Hz]"; dmp "Dämpfung in [kg/s]"; unc_bl "Rückschlag des Aktuators (Backlash) in [rad]"; unc_scale "Skalenfehler in [-]"; unc_off "Versatz (Offset) in [rad]"; siB_0 "Startwert Ruderwinkel in [rad]"; d_siB_0 "Startwert Ruderwinkelgeschwindigkeiten in [rad/s]"
      mask DialogControl ParameterGroupVar Prompt: Limitierungen
      mask DialogControl Container3 Prompt: Dynamik
      mask DialogControl Container4 Prompt: Aktuatorfehler
      mask DialogControl Container5 Prompt: Startwerte
  Rudder1 : Subsystem  mask{siB_max=siB_max, siB_min=siB_min, d_siB_max=d_siB_max, d_siB_min=d_siB_min, dd_siB_max=dd_siB_max, dd_siB_min=dd_siB_min, omega=act_omega, dmp=act_dmp, unc_bl=unc_act_bl, unc_scale=unc_act_scale, unc_off=unc_act_off, siB_0=siB_0, d_siB_0=d_siB_0}
      mask prompts: siB_max "Obere Limitierung des Ruderstellwinkels in [rad]"; siB_min "Untere Limitierung des Ruderstellwinkels in [rad]"; d_siB_max "Obere Limitierung der Ruderstellwinkelgeschwindigkeit in [rad/s]"; d_siB_min "Untere Limitierung der Ruderstellwinkelgeschwindigkeit in [rad/s]"; dd_siB_max "Obere Limitierung der Ruderstellwinkelbeschleunigung in [rad/s^2]"; dd_siB_min "Untere Limitierung der Ruderstellwinkelbeschleunigung in [rad/s^2]"; omega "Eckfrequenz in [Hz]"; dmp "Dämpfung in [kg/s]"; unc_bl "Rückschlag des Aktuators (Backlash) in [rad]"; unc_scale "Skalenfehler in [-]"; unc_off "Versatz (Offset) in [rad]"; siB_0 "Startwert Ruderwinkel in [rad]"; d_siB_0 "Startwert Ruderwinkelgeschwindigkeiten in [rad/s]"
      mask DialogControl ParameterGroupVar Prompt: Limitierungen
      mask DialogControl Container3 Prompt: Dynamik
      mask DialogControl Container4 Prompt: Aktuatorfehler
      mask DialogControl Container5 Prompt: Startwerte
  Rudder2 : Subsystem  mask{siB_max=siB_max, siB_min=siB_min, d_siB_max=d_siB_max, d_siB_min=d_siB_min, dd_siB_max=dd_siB_max, dd_siB_min=dd_siB_min, omega=act_omega, dmp=act_dmp, unc_bl=unc_act_bl, unc_scale=unc_act_scale, unc_off=unc_act_off, siB_0=siB_0, d_siB_0=d_siB_0}
      mask prompts: siB_max "Obere Limitierung des Ruderstellwinkels in [rad]"; siB_min "Untere Limitierung des Ruderstellwinkels in [rad]"; d_siB_max "Obere Limitierung der Ruderstellwinkelgeschwindigkeit in [rad/s]"; d_siB_min "Untere Limitierung der Ruderstellwinkelgeschwindigkeit in [rad/s]"; dd_siB_max "Obere Limitierung der Ruderstellwinkelbeschleunigung in [rad/s^2]"; dd_siB_min "Untere Limitierung der Ruderstellwinkelbeschleunigung in [rad/s^2]"; omega "Eckfrequenz in [Hz]"; dmp "Dämpfung in [kg/s]"; unc_bl "Rückschlag des Aktuators (Backlash) in [rad]"; unc_scale "Skalenfehler in [-]"; unc_off "Versatz (Offset) in [rad]"; siB_0 "Startwert Ruderwinkel in [rad]"; d_siB_0 "Startwert Ruderwinkelgeschwindigkeiten in [rad/s]"
      mask DialogControl ParameterGroupVar Prompt: Limitierungen
      mask DialogControl Container3 Prompt: Dynamik
      mask DialogControl Container4 Prompt: Aktuatorfehler
      mask DialogControl Container5 Prompt: Startwerte
  Rudder3 : Subsystem  mask{siB_max=siB_max, siB_min=siB_min, d_siB_max=d_siB_max, d_siB_min=d_siB_min, dd_siB_max=dd_siB_max, dd_siB_min=dd_siB_min, omega=act_omega, dmp=act_dmp, unc_bl=unc_act_bl, unc_scale=unc_act_scale, unc_off=unc_act_off, siB_0=siB_0, d_siB_0=d_siB_0}
      mask prompts: siB_max "Obere Limitierung des Ruderstellwinkels in [rad]"; siB_min "Untere Limitierung des Ruderstellwinkels in [rad]"; d_siB_max "Obere Limitierung der Ruderstellwinkelgeschwindigkeit in [rad/s]"; d_siB_min "Untere Limitierung der Ruderstellwinkelgeschwindigkeit in [rad/s]"; dd_siB_max "Obere Limitierung der Ruderstellwinkelbeschleunigung in [rad/s^2]"; dd_siB_min "Untere Limitierung der Ruderstellwinkelbeschleunigung in [rad/s^2]"; omega "Eckfrequenz in [Hz]"; dmp "Dämpfung in [kg/s]"; unc_bl "Rückschlag des Aktuators (Backlash) in [rad]"; unc_scale "Skalenfehler in [-]"; unc_off "Versatz (Offset) in [rad]"; siB_0 "Startwert Ruderwinkel in [rad]"; d_siB_0 "Startwert Ruderwinkelgeschwindigkeiten in [rad/s]"
      mask DialogControl ParameterGroupVar Prompt: Limitierungen
      mask DialogControl Container3 Prompt: Dynamik
      mask DialogControl Container4 Prompt: Aktuatorfehler
      mask DialogControl Container5 Prompt: Startwerte
  Switch : Switch  Criteria=u2 > Threshold
  Vector Concatenate1 : Concatenate  NumInputs=4
  Vector Concatenate2 : Concatenate  NumInputs=4
  Vector Concatenate3 : Concatenate  NumInputs=4
  control_allocation : Subsystem
  fin : Outport  VectorParamsAs1DForOutWhenUnconnected=off
  wires:
  [d_siB3] -> Vector Concatenate2/3
  Demux/4 -> Rudder3/1(siB_c)
  Rudder2/2(d_siB) -> [d_siB3]
  Rudder3/1(siB) -> Vector Concatenate1/4
  Rudder1/2(d_siB) -> [d_siB2]
  Rudder2/1(siB) -> Vector Concatenate1/3
  [d_siB4] -> Vector Concatenate2/4
  [d_siB1] -> Vector Concatenate2/1
  Bus Selector/1 -> Switch/3, Demux/1  "<siB_cmd>"
  [d_siB2] -> Vector Concatenate2/2
  Constant7/1 -> Rudder1/2(tRRR), Rudder3/2(tRRR), Rudder2/2(tRRR), Rudder/2(tRRR)
  [dd_siB2] -> Vector Concatenate3/2
  Demux/3 -> Rudder2/1(siB_c)
  Rudder3/2(d_siB) -> [d_siB4]
  Demux/1 -> Rudder/1(siB_c)
  [dd_siB4] -> Vector Concatenate3/4
  [dd_siB3] -> Vector Concatenate3/3
  cmd/1 -> Bus Selector/1
  [dd_siB1] -> Vector Concatenate3/1
  Rudder1/1(siB) -> Vector Concatenate1/2
  Rudder1/3(dd_siB) -> [dd_siB2]
  Rudder3/3(dd_siB) -> [dd_siB4]
  Rudder/2(d_siB) -> [d_siB1]
  Rudder2/3(dd_siB) -> [dd_siB3]
  Demux/2 -> Rudder1/1(siB_c)
  Rudder/3(dd_siB) -> [dd_siB1]
  Rudder/1(siB) -> Vector Concatenate1/1
  Bus Creator3/1 -> fin/1  "fin_bus"
  Switch/1 -> Bus Creator3/1, control_allocation/1(siB)  "siB"
  Vector Concatenate2/1 -> control_allocation/2(d_siB), Bus Creator3/7  "d_siB"
  Vector Concatenate3/1 -> Bus Creator3/6, control_allocation/3(dd_siB)  "dd_siB"
  control_allocation/1(Tr3r4) -> Bus Creator3/2
  control_allocation/2(finB) -> Bus Creator3/3
  control_allocation/3(d_finB) -> Bus Creator3/4
  control_allocation/4(dd_finB) -> Bus Creator3/5
  Vector Concatenate1/1 -> Switch/1  "siB"
  Constant/1 -> Switch/2

== system PIL_NO_RPI_new/Non-linear Flight Dynamic Model1/GRM_Airframe/forces_moments ==
  aero : Inport
  motion_kin : Inport  Port=2
  grav : Inport  Port=3
  prp : Inport  Port=4
  Add : Sum  Inputs=+++
  Add1 : Sum
  Bus Creator : BusCreator  Inputs=2
  Bus Selector : BusSelector  OutputSignals=FBAB,MBAB
  Bus Selector1 : BusSelector  OutputSignals=TGB
  Bus Selector2 : BusSelector  OutputSignals=FBGG
  Bus Selector3 : BusSelector  OutputSignals=FBPB,MBPB
  Math Function : Math  Operator=transpose  SignedPower=on  SaturateOnIntegerOverflow=on
  Product : Product  Multiplication=Matrix(*)
  for_mom_bus : Outport  VectorParamsAs1DForOutWhenUnconnected=off
  wires:
  Bus Selector/1 -> Add/1  "<FBAB>"
  Bus Selector2/1 -> Product/2  "<FBGG>"
  Bus Selector1/1 -> Math Function/1  "<TGB>"
  Math Function/1 -> Product/1  "TBG"
  aero/1 -> Bus Selector/1
  Product/1 -> Add/2  "FBGB"
  prp/1 -> Bus Selector3/1
  motion_kin/1 -> Bus Selector1/1
  Add/1 -> Bus Creator/1  "FBTB"
  grav/1 -> Bus Selector2/1
  Add1/1 -> Bus Creator/2  "MBTB"
  Bus Selector/2 -> Add1/1  "<MBAB>"
  Bus Selector3/1 -> Add/3  "<FBPB>"
  Bus Creator/1 -> for_mom_bus/1  "for_mom_bus"
  Bus Selector3/2 -> Add1/2  "<MBPB>"

== system PIL_NO_RPI_new/Non-linear Flight Dynamic Model1/GRM_Airframe/gravity ==
  env : Inport
  wab : Inport  Port=2
  Bus Creator3 : BusCreator  Inputs=1
  Bus Selector : BusSelector  OutputSignals=gBG,atm_bus.atm_stat_bus.hBE
  Bus Selector1 : BusSelector  OutputSignals=mB
  Product : Product
  launch_rail : Subsystem
  grav : Outport  VectorParamsAs1DForOutWhenUnconnected=off
  wires:
  launch_rail/1(gBG) -> Product/1
  Bus Selector/2 -> launch_rail/2(hBE)  "<hBE>"
  Bus Selector/1 -> launch_rail/1(gBG_c)  "<gBG>"
  Product/1 -> Bus Creator3/1  "FBGG"
  Bus Creator3/1 -> grav/1  "grav_bus"
  wab/1 -> Bus Selector1/1
  Bus Selector1/1 -> Product/2  "<mB>"
  env/1 -> Bus Selector/1

== system PIL_NO_RPI_new/Non-linear Flight Dynamic Model1/GRM_Airframe/input ==
  siB_cmd : Inport
  Bus Creator2 : BusCreator  Inputs=1
  cmd_bus : Outport  VectorParamsAs1DForOutWhenUnconnected=off
  wires:
  siB_cmd/1 -> Bus Creator2/1
  Bus Creator2/1 -> cmd_bus/1  "cmd_bus"

== system PIL_NO_RPI_new/Non-linear Flight Dynamic Model1/GRM_Airframe/motion_kinematics ==
  flight_dyn : Inport
  Bus Creator : BusCreator  Inputs=7
  Bus Selector : BusSelector  OutputSignals=lat,lon,qIB
  calc_motion_kinematics : Subsystem
  motion_kin : Outport  VectorParamsAs1DForOutWhenUnconnected=off
  wires:
  flight_dyn/1 -> Bus Selector/1
  Bus Creator/1 -> motion_kin/1  "motion_kin_bus"
  Bus Selector/1 -> calc_motion_kinematics/1(lat)  "<lat>"
  Bus Selector/2 -> calc_motion_kinematics/2(lon)  "<lon>"
  Bus Selector/3 -> calc_motion_kinematics/3(qIB)  "<qIB>"
  calc_motion_kinematics/1(wIEE) -> Bus Creator/1
  calc_motion_kinematics/2(TIE) -> Bus Creator/2
  calc_motion_kinematics/3(TEB) -> Bus Creator/3
  calc_motion_kinematics/4(TGB) -> Bus Creator/4
  calc_motion_kinematics/5(TEG) -> Bus Creator/5
  calc_motion_kinematics/6(wEGG) -> Bus Creator/6
  calc_motion_kinematics/7(TIB) -> Bus Creator/7

== system PIL_NO_RPI_new/Non-linear Flight Dynamic Model1/GRM_Airframe/propulsion ==
  env_glbl : Inport
  wab : Inport  Port=2
  Bus Creator1 : BusCreator  Inputs=2
  prp_look_up : Subsystem
  prp_uncertainty : Subsystem
  prp : Outport  VectorParamsAs1DForOutWhenUnconnected=off
  wires:
  Bus Creator1/1 -> prp/1  "prp_bus"
  prp_look_up/1(FBPM) -> prp_uncertainty/1(FBPM)
  env_glbl/1 -> prp_look_up/1(env_glbl_bus)
  prp_uncertainty/2(MBPB) -> Bus Creator1/2
  prp_uncertainty/1(FBPB) -> Bus Creator1/1
  wab/1 -> prp_uncertainty/2(wab)

== system PIL_NO_RPI_new/Non-linear Flight Dynamic Model1/GRM_Airframe/rb_eom ==
  mot_kin : Inport
  for_mom : Inport  Port=2
  wab : Inport  Port=3
  Bus Creator : BusCreator  Inputs=16
  calc_bus_flight_dyn_bus_entries : Subsystem
  eom_6dof : Subsystem
  flight_dyn : Outport  VectorParamsAs1DForOutWhenUnconnected=off
  wires:
  mot_kin/1 -> calc_bus_flight_dyn_bus_entries/1(mot_kin)
  calc_bus_flight_dyn_bus_entries/1(aBIB) -> Bus Creator/1
  calc_bus_flight_dyn_bus_entries/2(lon) -> Bus Creator/2
  calc_bus_flight_dyn_bus_entries/3(lat) -> Bus Creator/3
  calc_bus_flight_dyn_bus_entries/4(hBE) -> Bus Creator/4
  calc_bus_flight_dyn_bus_entries/5(vBII) -> Bus Creator/5
  calc_bus_flight_dyn_bus_entries/6(qIB) -> Bus Creator/6
  calc_bus_flight_dyn_bus_entries/7(wBIB) -> Bus Creator/7
  calc_bus_flight_dyn_bus_entries/8(d_wBIB) -> Bus Creator/8
  calc_bus_flight_dyn_bus_entries/9(d_vBII) -> Bus Creator/9
  Bus Creator/1 -> flight_dyn/1  "flight_dyn_bus"
  for_mom/1 -> eom_6dof/1(for_mom)
  wab/1 -> eom_6dof/2(wab)
  eom_6dof/1(eom) -> calc_bus_flight_dyn_bus_entries/2(eom)
  calc_bus_flight_dyn_bus_entries/10(pBII) -> Bus Creator/10
  calc_bus_flight_dyn_bus_entries/11(euIB) -> Bus Creator/11
  calc_bus_flight_dyn_bus_entries/12(vBIB) -> Bus Creator/12
  calc_bus_flight_dyn_bus_entries/13(qGB) -> Bus Creator/13
  calc_bus_flight_dyn_bus_entries/14(euGB) -> Bus Creator/14
  calc_bus_flight_dyn_bus_entries/15(euBG) -> Bus Creator/15
  calc_bus_flight_dyn_bus_entries/16(pBLG) -> Bus Creator/16

== system PIL_NO_RPI_new/Non-linear Flight Dynamic Model1/GRM_Airframe/stream_flow ==
  flight_dyn : Inport
  motion_kin : Inport  Port=2
  env : Inport  Port=3
  Bus Selector1 : BusSelector  OutputSignals=atm_bus.atm_stat_bus.rho,atm_bus.atm_stat_bus.sos,atm_bus.atm_stat_bus.hBE
  Bus Selector2 : BusSelector  OutputSignals=vBII,pBII,wBIB
  Bus Selector3 : BusSelector  OutputSignals=TIB,wIEE,TIE
  calc_stream_flow : Subsystem
  str_flow : Outport  VectorParamsAs1DForOutWhenUnconnected=off
  wires:
  motion_kin/1 -> Bus Selector3/1
  flight_dyn/1 -> Bus Selector2/1
  env/1 -> Bus Selector1/1
  Bus Selector3/1 -> calc_stream_flow/1(TIB)  "<TIB>"
  Bus Selector3/2 -> calc_stream_flow/2(wIEE)  "<wIEE>"
  Bus Selector3/3 -> calc_stream_flow/3(TIE)  "<TIE>"
  Bus Selector2/1 -> calc_stream_flow/4(VBII)  "<vBII>"
  Bus Selector2/3 -> calc_stream_flow/6(wBIB)  "<wBIB>"
  Bus Selector1/1 -> calc_stream_flow/7(rho)  "<rho>"
  Bus Selector1/2 -> calc_stream_flow/8(sos)  "<sos>"
  Bus Selector1/3 -> calc_stream_flow/9(hBE)  "<hBE>"
  calc_stream_flow/1(str_flow) -> str_flow/1
  Bus Selector2/2 -> calc_stream_flow/5(pBII)  "<pBII>"

== system PIL_NO_RPI_new/Non-linear Flight Dynamic Model1/GRM_Airframe/weight_and_balance ==
  env_glb : Inport
  Bus Creator1 : BusCreator  Inputs=3
  Bus Selector2 : BusSelector  OutputSignals=T_sim_glbl,T_sim_lnch
  Subtract : Sum  Inputs=+-
  center_of_gravity : Subsystem
  mass : Subsystem
  mass_uncertainty : Subsystem
  moi : Subsystem
  wab : Outport  VectorParamsAs1DForOutWhenUnconnected=off
  wires:
  Bus Selector2/2 -> Subtract/2  "<T_sim_lnch>"
  Bus Selector2/1 -> Subtract/1  "<T_sim_glbl>"
  env_glb/1 -> Bus Selector2/1
  Bus Creator1/1 -> wab/1  "wab_bus"
  center_of_gravity/1(pBPB) -> moi/1(pBPB), Bus Creator1/2
  moi/1(JBBB) -> Bus Creator1/3
  mass/2(mM) -> moi/2(mM), center_of_gravity/2(mM)
  mass_uncertainty/1(mB) -> center_of_gravity/1(mB), Bus Creator1/1
  mass/1(mB_c) -> mass_uncertainty/1(mB_c)
  Subtract/1 -> mass/1(sim_time_launch)

== system PIL_NO_RPI_new/Non-linear Flight Dynamic Model1/Stop-Condition/Compare To Constant ==
  u : Inport
  Compare : RelationalOperator  Operator=>  OutDataTypeStr=boolean  RndMeth=Nearest  InputSameDT=on
  Constant : Constant  DisableCoverage=on  Value=const  OutDataTypeStr=Inherit: Inherit via back propagation
  y : Outport
  wires:
  u/1 -> Compare/1
  Constant/1 -> Compare/2
  Compare/1 -> y/1

== system PIL_NO_RPI_new/Non-linear Flight Dynamic Model1/Stop-Condition/Compare To Constant1 ==
  u : Inport
  Compare : RelationalOperator  Operator=>  OutDataTypeStr=boolean  RndMeth=Nearest  InputSameDT=on
  Constant : Constant  DisableCoverage=on  Value=const  OutDataTypeStr=Inherit: Inherit via back propagation
  y : Outport
  wires:
  Compare/1 -> y/1
  Constant/1 -> Compare/2
  u/1 -> Compare/1
